simulink model "PD_ctl_sim"  (R2023a)
settings: Solver=VariableStepAuto  StartTime=0.0  StopTime=10.0  RelTol=1e-3
values from neighbouring files (symbols this model uses):
  cong = [1, 1, 1]*0.5/3600*d2r    [PD_ctl_m.m]
  fei1 = [10, 10, 30]'*d2r    [PD_ctl_m.m]
  Kd = [2*wnx*1.25/0.515*2, 2*wny*9.65/3.18, 2*wnz*9.65/1.59*2]*sqrt(0.6)    [PD_ctl_m.m]
  Kp = [1.25/0.515*wnx^2*0.6, 9.65/3.18*wny^2*0.6, 9.65/1.59*wnz^2*0.6]*2    [PD_ctl_m.m]
  Noig = [1, 1, 1]*1/3*5*10^(-5)*d2r    [PD_ctl_m.m]
  Q0 = [Q1 Q2 Q3]    [PD_ctl_m.m]
  Q00 = cos(fei0(1)/2)*cos(fei0(2)/2)*cos(fei0(3)/2) + sin(fei0(1)/2)*sin(fei0(2)/2)*sin(fei0(3)/2)    [PD_ctl_m.m]
  Wio = [0 -2*pi/5431.184 0]'    [PD_ctl_m.m]
undefined symbols (not defined in the file or in its folder): HBO, invIB, Qt, Tscontrol
libraries: sharedutil x1
settings Model: Creator=LuBin  LastModifiedBy=bin.lu
settings SolverCC: AlgebraicLoopSolver=TrustRegion
settings DebuggingCC: UnconnectedInputMsg=warning  UnconnectedOutputMsg=warning  UnconnectedLineMsg=warning
settings ModelReferenceCC: EnableRefExpFcnMdlSchedulingChecks=on
settings RTWCC: DLArmComputeVersion=19.05

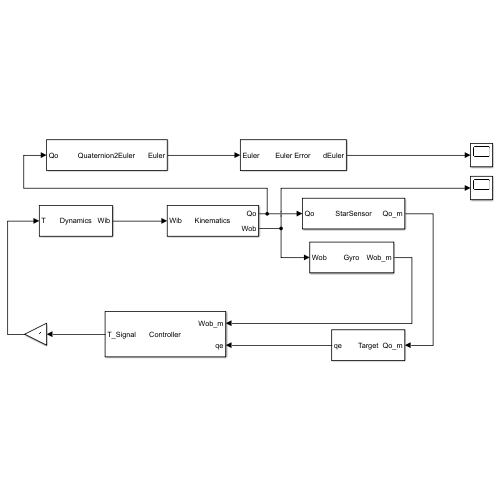
[thumbnail: Simulink's stored preview of the top-level diagram]
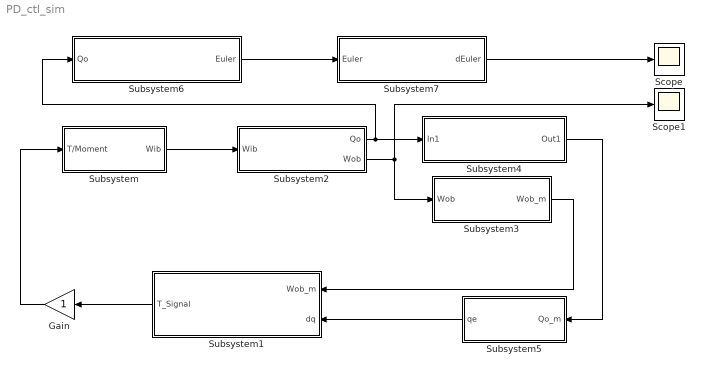
== system PD_ctl_sim ==
  Gain : Gain
  Scope : Scope
  Scope1 : Scope
  Subsystem : Subsystem
      mask Display:
      | disp('Dynamics')
      | port_label('input', 1, 'T')
      | port_label('output', 1, 'Wib')
  Subsystem1 : Subsystem
      mask Display:
      | disp('Controller')
      | port_label('input', 1, 'Wob_m')
      | port_label('input', 2, 'qe')
      | port_label('output', 1, 'T_Signal')
  Subsystem2 : Subsystem
      mask Display:
      | disp('Kinematics')
      | port_label('input', 1, 'Wib')
      | port_label('output', 1, 'Qo')
      | port_label('output', 2, 'Wob')
  Subsystem3 : Subsystem
      mask Display:
      | disp('Gyro')
      | port_label('input', 1, 'Wob')
      | port_label('output', 1, 'Wob_m')
  Subsystem4 : Subsystem
      mask Display:
      | disp('StarSensor')
      | port_label('input', 1, 'Qo')
      | port_label('output', 1, 'Qo_m')
  Subsystem5 : Subsystem
      mask Display:
      | disp('Target')
      | port_label('input', 1, 'Qo_m')
      | port_label('output', 1, 'qe')
  Subsystem6 : Subsystem
      mask Display:
      | disp('Quaternion2Euler')
      | port_label('input', 1, 'Qo')
      | port_label('output', 1, 'Euler')
  Subsystem7 : Subsystem
      mask Display:
      | disp('Euler Error')
      | port_label('input', 1, 'Euler')
      | port_label('output', 1, 'dEuler')
  wires:
  Subsystem/1(Wib) -> Subsystem2/1(Wib)
  Subsystem2/1(Qo) -> Subsystem6/1(Qo), Subsystem4/1(In1)
  Subsystem2/2(Wob) -> Subsystem3/1(Wob), Scope1/1
  Subsystem4/1(Out1) -> Subsystem5/1(Qo_m)
  Subsystem5/1(qe) -> Subsystem1/2(dq)
  Subsystem1/1(T_Signal) -> Gain/1
  Gain/1 -> Subsystem/1(T/Moment)
  Subsystem6/1(Euler) -> Subsystem7/1(Euler)
  Subsystem7/1(dEuler) -> Scope/1
  Subsystem3/1(Wob_m) -> Subsystem1/1(Wob_m)

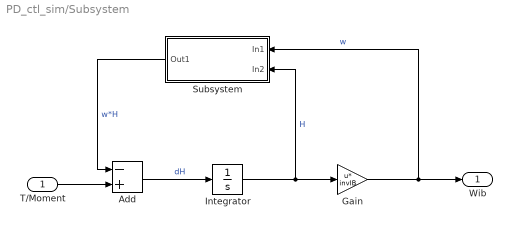
== system PD_ctl_sim/Subsystem ==
  T/Moment : Inport
  Add : Sum  Inputs=-+
  Gain : Gain  Gain=invIB  Multiplication=Matrix(u*K)
  Integrator : Integrator  InitialCondition=HBO
  Subsystem : Subsystem
      mask Display:
      | disp('Cross \nProduct')
      | port_label('input', 1, 'X')
      | port_label('input', 2, 'Y')
      | port_label('output', 1, 'X*Y')
  Wib : Outport
  wires:
  T/Moment/1 -> Add/2
  Add/1 -> Integrator/1  "dH"
  Integrator/1 -> Subsystem/2(In2), Gain/1  "H"
  Gain/1 -> Subsystem/1(In1), Wib/1  "w"
  Subsystem/1(Out1) -> Add/1  "w*H"

== system PD_ctl_sim/Subsystem1 ==
  Wob_m : Inport
  dq : Inport  Port=2
  Add : Sum  Inputs=--
  Gain : Gain  Gain=Kd
  Gain1 : Gain  Gain=Kp
  T_Signal : Outport
  wires:
  Gain1/1 -> Add/2
  Gain/1 -> Add/1
  Add/1 -> T_Signal/1
  dq/1 -> Gain1/1
  Wob_m/1 -> Gain/1

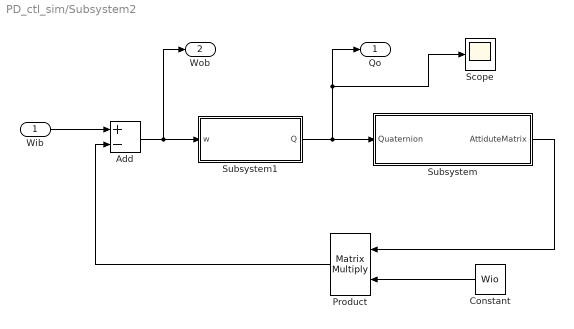
== system PD_ctl_sim/Subsystem2 ==
  Wib : Inport
  Add : Sum  Inputs=+-
  Constant : Constant  Value=Wio
  Product : Product  Multiplication=Matrix(*)
  Scope : Scope
  Subsystem : Subsystem
      mask Display:
      | disp('Quaternion2 \nAttitudeMatrix')
      | port_label('input', 1, 'Qua')
      | port_label('output', 1, 'Matrix')
  Subsystem1 : Subsystem
      mask Display:
      | disp('Quaternion \nSolve Model')
      | port_label('input', 1, 'wob')
      | port_label('output', 1, 'Q')
  Qo : Outport
  Wob : Outport  Port=2
  wires:
  Constant/1 -> Product/2
  Wib/1 -> Add/1
  Add/1 -> Wob/1, Subsystem1/1(w)
  Subsystem1/1(Q) -> Scope/1, Qo/1, Subsystem/1(Quaternion)
  Subsystem/1(AttiduteMatrix) -> Product/1
  Product/1 -> Add/2

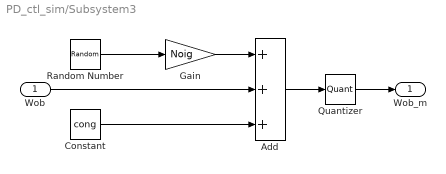
== system PD_ctl_sim/Subsystem3 ==
  Wob : Inport
  Add : Sum  Inputs=+++
  Constant : Constant  Value=cong
  Gain : Gain  Gain=Noig
  Quantizer : Quantizer  QuantizationInterval=Gyquan
  Random Number : RandomNumber  Mean=[0, 0, 0]  Variance=[1, 1, 1]  Seed=fix(abs(100000*rand([3,1])))  SampleTime=Tscontrol
  Wob_m : Outport
  wires:
  Random Number/1 -> Gain/1
  Gain/1 -> Add/1
  Wob/1 -> Add/2
  Constant/1 -> Add/3
  Add/1 -> Quantizer/1
  Quantizer/1 -> Wob_m/1

== system PD_ctl_sim/Subsystem4 ==
  In1 : Inport
  Out1 : Outport
  wires:
  In1/1 -> Out1/1

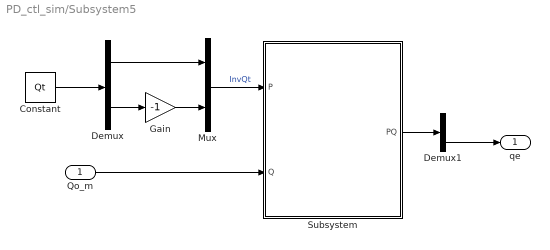
== system PD_ctl_sim/Subsystem5 ==
  Qo_m : Inport
  Constant : Constant  Value=Qt
  Demux : Demux  Outputs=[1 3]
  Demux1 : Demux  Outputs=[1 3]
  Gain : Gain  Gain=-1
  Mux : Mux  Inputs=[1 3]
  Subsystem : Subsystem
      mask Display:
      | disp('InterQ Multiply')
      | port_label('input', 1, 'P')
      | port_label('input', 2, 'Q')
      | port_label('output', 1, 'PQ')
  qe : Outport
  wires:
  Qo_m/1 -> Subsystem/2(Q)
  Constant/1 -> Demux/1
  Gain/1 -> Mux/2
  Demux/2 -> Gain/1
  Demux/1 -> Mux/1
  Mux/1 -> Subsystem/1(P)  "InvQt"
  Demux1/2 -> qe/1
  Subsystem/1(PQ) -> Demux1/1

== system PD_ctl_sim/Subsystem6 ==
  Qo : Inport
  Mux : Mux  Inputs=3
  Phi : MATLAB Function  TreatAsAtomicUnit=on
  Psi : MATLAB Function  TreatAsAtomicUnit=on
  Theta : MATLAB Function  TreatAsAtomicUnit=on
  Euler : Outport
  wires:
  Mux/1 -> Euler/1
  Theta/1(y) -> Mux/2
  Phi/1(y) -> Mux/1
  Psi/1(y) -> Mux/3
  Qo/1 -> Psi/1(u), Phi/1(u), Theta/1(u)

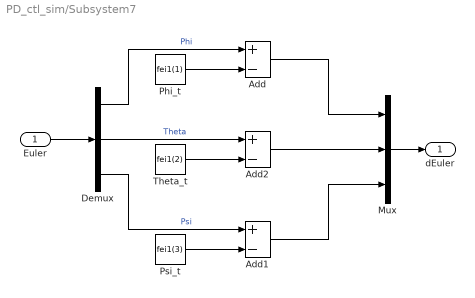
== system PD_ctl_sim/Subsystem7 ==
  Euler : Inport
  Add : Sum  Inputs=+-
  Add1 : Sum  Inputs=+-
  Add2 : Sum  Inputs=+-
  Demux : Demux  Outputs=3
  Mux : Mux  Inputs=3
  Phi_t : Constant  Value=fei1(1)
  Psi_t : Constant  Value=fei1(3)
  Theta_t : Constant  Value=fei1(2)
  dEuler : Outport
  wires:
  Phi_t/1 -> Add/2
  Theta_t/1 -> Add2/2
  Psi_t/1 -> Add1/2
  Euler/1 -> Demux/1
  Demux/1 -> Add/1  "Phi"
  Demux/2 -> Add2/1  "Theta"
  Demux/3 -> Add1/1  "Psi"
  Mux/1 -> dEuler/1
  Add2/1 -> Mux/2
  Add/1 -> Mux/1
  Add1/1 -> Mux/3

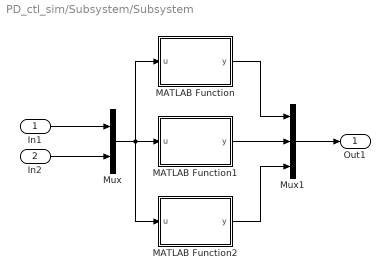
== system PD_ctl_sim/Subsystem/Subsystem ==
  In1 : Inport
  In2 : Inport  Port=2
  MATLAB Function : MATLAB Function  TreatAsAtomicUnit=on
  MATLAB Function1 : MATLAB Function  TreatAsAtomicUnit=on
  MATLAB Function2 : MATLAB Function  TreatAsAtomicUnit=on
  Mux : Mux  Inputs=[3 3]
  Mux1 : Mux  Inputs=[1 1 1]
  Out1 : Outport
  wires:
  In1/1 -> Mux/1
  In2/1 -> Mux/2
  Mux/1 -> MATLAB Function2/1(u), MATLAB Function/1(u), MATLAB Function1/1(u)
  MATLAB Function/1(y) -> Mux1/1
  MATLAB Function1/1(y) -> Mux1/2
  MATLAB Function2/1(y) -> Mux1/3
  Mux1/1 -> Out1/1

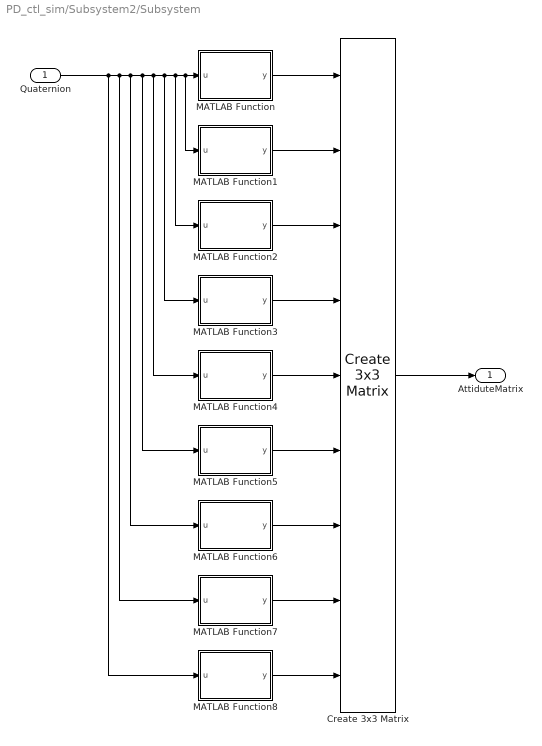
== system PD_ctl_sim/Subsystem2/Subsystem ==
  Quaternion : Inport
  Create 3x3 Matrix : sharedutil/Create 3x3 Matrix  aMode=aMode
  MATLAB Function : MATLAB Function  TreatAsAtomicUnit=on
  MATLAB Function1 : MATLAB Function  TreatAsAtomicUnit=on
  MATLAB Function2 : MATLAB Function  TreatAsAtomicUnit=on
  MATLAB Function3 : MATLAB Function  TreatAsAtomicUnit=on
  MATLAB Function4 : MATLAB Function  TreatAsAtomicUnit=on
  MATLAB Function5 : MATLAB Function  TreatAsAtomicUnit=on
  MATLAB Function6 : MATLAB Function  TreatAsAtomicUnit=on
  MATLAB Function7 : MATLAB Function  TreatAsAtomicUnit=on
  MATLAB Function8 : MATLAB Function  TreatAsAtomicUnit=on
  AttiduteMatrix : Outport
  wires:
  Create 3x3 Matrix/1 -> AttiduteMatrix/1
  Quaternion/1 -> MATLAB Function8/1(u), MATLAB Function7/1(u), MATLAB Function6/1(u), MATLAB Function5/1(u), MATLAB Function4/1(u), MATLAB Function3/1(u), MATLAB Function2/1(u), MATLAB Function1/1(u), MATLAB Function/1(u)
  MATLAB Function/1(y) -> Create 3x3 Matrix/1
  MATLAB Function1/1(y) -> Create 3x3 Matrix/2
  MATLAB Function2/1(y) -> Create 3x3 Matrix/3
  MATLAB Function3/1(y) -> Create 3x3 Matrix/4
  MATLAB Function4/1(y) -> Create 3x3 Matrix/5
  MATLAB Function5/1(y) -> Create 3x3 Matrix/6
  MATLAB Function6/1(y) -> Create 3x3 Matrix/7
  MATLAB Function7/1(y) -> Create 3x3 Matrix/8
  MATLAB Function8/1(y) -> Create 3x3 Matrix/9

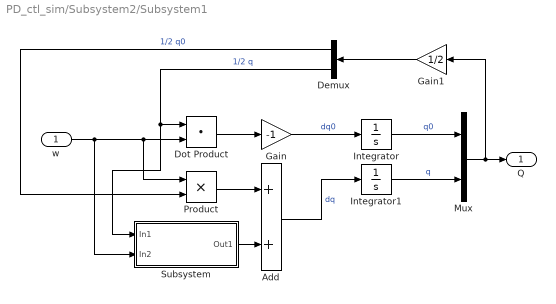
== system PD_ctl_sim/Subsystem2/Subsystem1 ==
  w : Inport
  Add : Sum
  Demux : Demux  Outputs=[1 3]
  Dot Product : DotProduct  OutDataTypeStr=Inherit: Inherit via internal rule
  Gain : Gain  Gain=-1
  Gain1 : Gain  Gain=1/2
  Integrator : Integrator  InitialCondition=Q00
  Integrator1 : Integrator  InitialCondition=Q0
  Mux : Mux  Inputs=[1 3]
  Product : Product
  Subsystem : Subsystem
      mask Display:
      | disp('Cross \nProduct')
      | port_label('input', 1, 'X')
      | port_label('input', 2, 'Y')
      | port_label('output', 1, 'X*Y')
  Q : Outport
  wires:
  Mux/1 -> Gain1/1, Q/1
  Add/1 -> Integrator1/1  "dq"
  Gain/1 -> Integrator/1  "dq0"
  Integrator/1 -> Mux/1  "q0"
  Integrator1/1 -> Mux/2  "q"
  Gain1/1 -> Demux/1
  Dot Product/1 -> Gain/1
  Product/1 -> Add/1
  Subsystem/1(Out1) -> Add/2
  w/1 -> Subsystem/2(In2), Product/1, Dot Product/2
  Demux/2 -> Subsystem/1(In1), Dot Product/1  "1/2 q"
  Demux/1 -> Product/2  "1/2 q0"

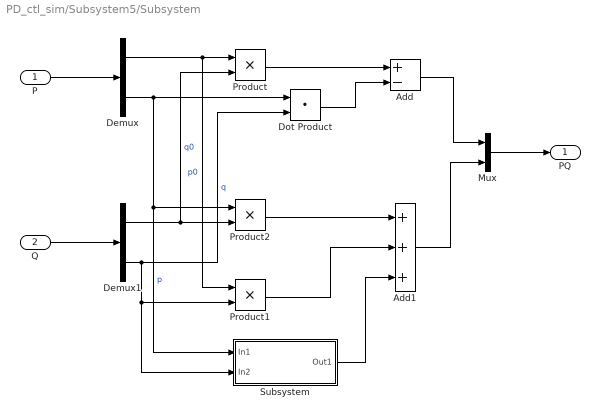
== system PD_ctl_sim/Subsystem5/Subsystem ==
  P : Inport
  Q : Inport  Port=2
  Add : Sum  Inputs=+-
  Add1 : Sum  Inputs=+++
  Demux : Demux  Outputs=[1 3]
  Demux1 : Demux  Outputs=[1 3]
  Dot Product : DotProduct  OutDataTypeStr=Inherit: Inherit via internal rule
  Mux : Mux  Inputs=[1 3]
  Product : Product
  Product1 : Product
  Product2 : Product
  Subsystem : Subsystem
      mask Display:
      | disp('Cross \nProduct')
      | port_label('input', 1, 'X')
      | port_label('input', 2, 'Y')
      | port_label('output', 1, 'X*Y')
  PQ : Outport
  wires:
  P/1 -> Demux/1
  Q/1 -> Demux1/1
  Mux/1 -> PQ/1
  Demux/1 -> Product1/1, Product/1  "p0"
  Demux1/1 -> Product2/2, Product/2  "q0"
  Demux/2 -> Dot Product/1, Subsystem/1(In1), Product2/1  "p"
  Demux1/2 -> Subsystem/2(In2), Product1/2, Dot Product/2  "q"
  Product/1 -> Add/1
  Dot Product/1 -> Add/2
  Product2/1 -> Add1/1
  Product1/1 -> Add1/2
  Subsystem/1(Out1) -> Add1/3
  Add/1 -> Mux/1
  Add1/1 -> Mux/2

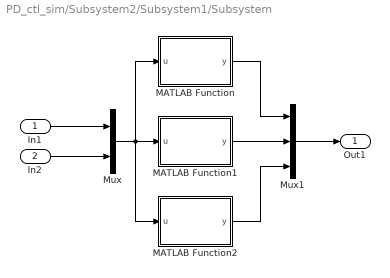
== system PD_ctl_sim/Subsystem2/Subsystem1/Subsystem ==
  In1 : Inport
  In2 : Inport  Port=2
  MATLAB Function : MATLAB Function  TreatAsAtomicUnit=on
  MATLAB Function1 : MATLAB Function  TreatAsAtomicUnit=on
  MATLAB Function2 : MATLAB Function  TreatAsAtomicUnit=on
  Mux : Mux  Inputs=[3 3]
  Mux1 : Mux  Inputs=[1 1 1]
  Out1 : Outport
  wires:
  In1/1 -> Mux/1
  In2/1 -> Mux/2
  Mux/1 -> MATLAB Function2/1(u), MATLAB Function/1(u), MATLAB Function1/1(u)
  MATLAB Function/1(y) -> Mux1/1
  MATLAB Function1/1(y) -> Mux1/2
  MATLAB Function2/1(y) -> Mux1/3
  Mux1/1 -> Out1/1

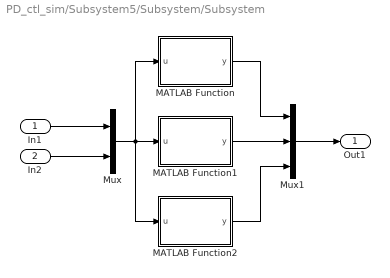
== system PD_ctl_sim/Subsystem5/Subsystem/Subsystem ==
  In1 : Inport
  In2 : Inport  Port=2
  MATLAB Function : MATLAB Function  TreatAsAtomicUnit=on
  MATLAB Function1 : MATLAB Function  TreatAsAtomicUnit=on
  MATLAB Function2 : MATLAB Function  TreatAsAtomicUnit=on
  Mux : Mux  Inputs=[3 3]
  Mux1 : Mux  Inputs=[1 1 1]
  Out1 : Outport
  wires:
  In1/1 -> Mux/1
  In2/1 -> Mux/2
  Mux/1 -> MATLAB Function2/1(u), MATLAB Function/1(u), MATLAB Function1/1(u)
  MATLAB Function/1(y) -> Mux1/1
  MATLAB Function1/1(y) -> Mux1/2
  MATLAB Function2/1(y) -> Mux1/3
  Mux1/1 -> Out1/1

== matlab function PD_ctl_sim/Subsystem2/Subsystem1/Subsystem/MATLAB Function2 ==
  data: u input; y output
function y = fcn(u)

y = u(1)*u(5) - u(2)*u(4);

== matlab function PD_ctl_sim/Subsystem5/Subsystem/Subsystem/MATLAB Function ==
  data: u input; y output
function y = fcn(u)

y = u(2)*u(6) - u(3)*u(5);

== matlab function PD_ctl_sim/Subsystem5/Subsystem/Subsystem/MATLAB Function1 ==
  data: u input; y output
function y = fcn(u)

y = u(3)*u(4) - u(1)*u(6);

== matlab function PD_ctl_sim/Subsystem5/Subsystem/Subsystem/MATLAB Function2 ==
  data: u input; y output
function y = fcn(u)

y = u(1)*u(5) - u(2)*u(4);

== matlab function PD_ctl_sim/Subsystem6/Phi ==
  data: u input; y output
function y = fcn(u)

y = atan(2*(u(1)*u(2) + u(3)*u(4))/(u(1)^2 - u(2)^2 - u(3)^2 + u(4)^2));

== matlab function PD_ctl_sim/Subsystem/Subsystem/MATLAB Function ==
  data: u input; y output
function y = fcn(u)

y = u(2)*u(6) - u(3)*u(5);

== matlab function PD_ctl_sim/Subsystem6/Theta ==
  data: u input; y output
function y = fcn(u)

y = asin(-2*(u(2)*u(4) - u(1)*u(3)));

== matlab function PD_ctl_sim/Subsystem6/Psi ==
  data: u input; y output
function y = fcn(u)

y = atan(2*(u(2)*u(3) + u(1)*u(4))/(u(1)^2 + u(2)^2 - u(3)^2 - u(4)^2));

== matlab function PD_ctl_sim/Subsystem/Subsystem/MATLAB Function2 ==
  data: u input; y output
function y = fcn(u)

y = u(1)*u(5) - u(2)*u(4);

== matlab function PD_ctl_sim/Subsystem2/Subsystem/MATLAB Function ==
  data: u input; y output
function y = fcn(u)

y = 1 - 2*(u(3)*u(3) + u(4)*u(4));

== matlab function PD_ctl_sim/Subsystem2/Subsystem/MATLAB Function1 ==
  data: u input; y output
function y = fcn(u)

y = 2*(u(2)*u(3) + u(1)*u(4));

== matlab function PD_ctl_sim/Subsystem2/Subsystem/MATLAB Function2 ==
  data: u input; y output
function y = fcn(u)

y = 2*(-u(1)*u(3) + u(2)*u(4));

== matlab function PD_ctl_sim/Subsystem2/Subsystem/MATLAB Function3 ==
  data: u input; y output
function y = fcn(u)

y = 2*(u(2)*u(3) - u(1)*u(4));

== matlab function PD_ctl_sim/Subsystem2/Subsystem/MATLAB Function4 ==
  data: u input; y output
function y = fcn(u)

y = 1 - 2*(u(2)*u(2) + u(4)*u(4));

== matlab function PD_ctl_sim/Subsystem2/Subsystem/MATLAB Function5 ==
  data: u input; y output
function y = fcn(u)

y = 2*(u(1)*u(2) + u(3)*u(4));

== matlab function PD_ctl_sim/Subsystem/Subsystem/MATLAB Function1 ==
  data: u input; y output
function y = fcn(u)

y = u(3)*u(4) - u(1)*u(6);

== matlab function PD_ctl_sim/Subsystem2/Subsystem/MATLAB Function6 ==
  data: u input; y output
function y = fcn(u)

y = 2*(u(1)*u(3) + u(2)*u(4));

== matlab function PD_ctl_sim/Subsystem2/Subsystem/MATLAB Function7 ==
  data: u input; y output
function y = fcn(u)

y = 2*(-u(1)*u(2) + u(3)*u(4));

== matlab function PD_ctl_sim/Subsystem2/Subsystem/MATLAB Function8 ==
  data: u input; y output
function y = fcn(u)

y = 1 - 2*(u(2)*u(2) + u(3)*u(3));

== matlab function PD_ctl_sim/Subsystem2/Subsystem1/Subsystem/MATLAB Function ==
  data: u input; y output
function y = fcn(u)

y = u(2)*u(6) - u(3)*u(5);

== matlab function PD_ctl_sim/Subsystem2/Subsystem1/Subsystem/MATLAB Function1 ==
  data: u input; y output
function y = fcn(u)

y = u(3)*u(4) - u(1)*u(6);
